simulink model "main_hexaglide_lin_alg_z"  (Simulink 7.8)
settings: Solver=ode45  StartTime=0.0  StopTime=50  RelTol=1e-3
values from neighbouring files (symbols this model uses):
  q = [z11;z12;z21;z22;z31;z32;phi11;phi12;phi21;phi22;phi31;phi32;theta11;theta12;theta21;theta22;theta31;theta32;X;Y;Z;phi;theta;psi;]    [environment.m]
settings Model: Creator=imac  LastModifiedBy=roberto
settings DebuggingCC: FcnCallInpInsideContextMsg=Use local settings

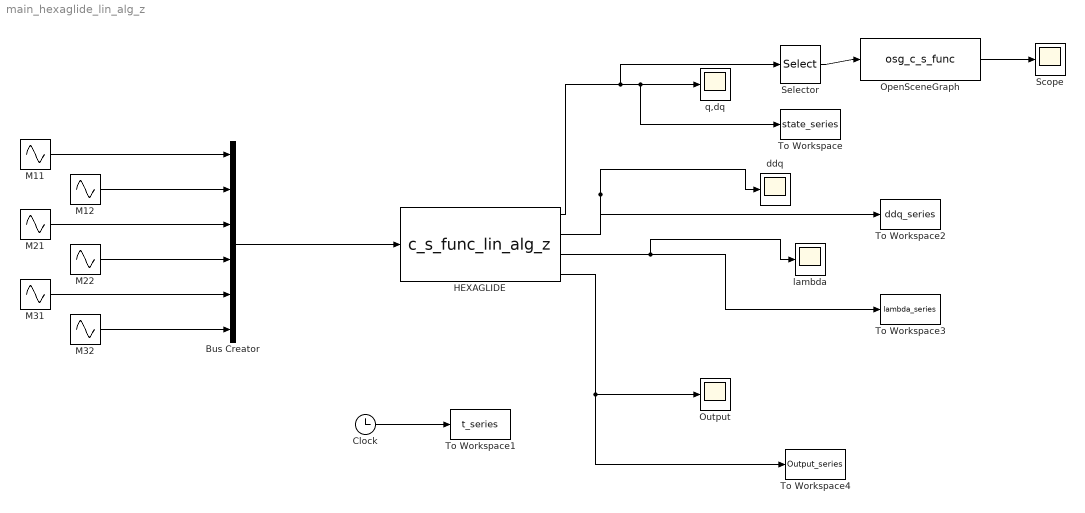
== system main_hexaglide_lin_alg_z ==
  Bus Creator : BusCreator  Inputs=6
  Clock : Clock
  HEXAGLIDE : S-Function  FunctionName=c_s_func_lin_alg_z  Parameters=q dq param  EnableBusSupport=off
      mask Type: S-function: mycsfunc
      mask Description: This is a S-function that does the continuous state space system.
      mask Display: disp('[M , Phi_q''] [ddq]\n[Phi_q , 0] [lambda]\n=\n [Q ] \n   [gamma] ');
  M11 : Sin  Description=FX  Amplitude=.2  Phase=pi/2  SampleTime=0
  M12 : Sin  Amplitude=-.2  Phase=pi/2  SampleTime=0
  M21 : Sin  Amplitude=.2  Phase=pi/2  SampleTime=0
  M22 : Sin  Amplitude=-.2  Phase=pi/2  SampleTime=0
  M31 : Sin  Amplitude=.2  Phase=pi/2  SampleTime=0
  M32 : Sin  Amplitude=-.2  Phase=pi/2  SampleTime=0
  OpenSceneGraph : S-Function  FunctionName=osg_c_s_func  EnableBusSupport=off
  Output : Scope
      settings: YMin=-70  YMax=20  SaveName=ScopeData3  SampleInput=on  SampleTime=0.01
  Scope : Scope
      settings: SaveName=ScopeData4
  Selector : Selector  InputPortWidth=2*length(q)  IndexOptions=Index vector (dialog)  Indices=1:1:length(q)  OutputSizes=1
  To Workspace : ToWorkspace  VariableName=state_series  SampleTime=0.01  SaveFormat=Array
  To Workspace1 : ToWorkspace  VariableName=t_series  SampleTime=0.01  SaveFormat=Array
  To Workspace2 : ToWorkspace  VariableName=ddq_series  SampleTime=0.01  SaveFormat=Array
  To Workspace3 : ToWorkspace  VariableName=lambda_series  SampleTime=0.01  SaveFormat=Array
  To Workspace4 : ToWorkspace  VariableName=Output_series  SampleTime=0.01  SaveFormat=Array
  ddq : Scope
      settings: YMin=-0.05  YMax=0.6  SampleInput=on  SampleTime=0.01
  lambda : Scope
      settings: TimeRange=5  YMin=274.2  YMax=275.7  SaveName=ScopeData2  SampleInput=on  SampleTime=0.01
  q,dq : Scope
      settings: YMin=-0.025  YMax=0.425  SampleInput=on  SampleTime=0.01
  wires:
  Clock/1 -> To Workspace1/1
  HEXAGLIDE/1 -> q,dq/1, To Workspace/1, Selector/1
  HEXAGLIDE/2 -> ddq/1, To Workspace2/1
  HEXAGLIDE/3 -> lambda/1, To Workspace3/1
  HEXAGLIDE/4 -> Output/1, To Workspace4/1
  Selector/1 -> OpenSceneGraph/1
  OpenSceneGraph/1 -> Scope/1
  Bus Creator/1 -> HEXAGLIDE/1
  M21/1 -> Bus Creator/3
  M31/1 -> Bus Creator/5
  M22/1 -> Bus Creator/4
  M32/1 -> Bus Creator/6
  M11/1 -> Bus Creator/1
  M12/1 -> Bus Creator/2
